simulink model "Milestone_2_Hardware"  (R2021a)
settings: Solver=FixedStepDiscrete  StartTime=0.0  StopTime=10  FixedStep=0.01  RelTol=1e-3  EnableMultiTasking=on
values from neighbouring files (symbols this model uses):
  ticksPerRot =     [robotParameters.m]
  wheelR =     [robotParameters.m]
undefined symbols (not defined in the file or in its folder): InputPWM, WheelSpeed
libraries: arduinolib x10, spsEdgeDetectorLib x2, pid_lib x2, mobileRoboticsTrainingLib x1
settings Model: SILPILModeSetting=veronly  ExtModeTrigDuration=2  Creator=Boitumelo  LastModifiedBy=brennannaidoo
settings OptimizationCC: EnhancedBackFolding=on  PassReuseOutputArgsAs=Individual arguments  ZeroExternalMemoryAtStartup=off  ZeroInternalMemoryAtStartup=off  MaxStackSize=64  OptimizeBlockOrder=speed  DifferentSizesBufferReuse=on  OptimizationCustomize=off  EfficientTunableParamExpr=on
settings DebuggingCC: ParameterTunabilityLossMsg=error
settings HardwareCC: ProdBitPerInt=16  ProdBitPerPointer=16  ProdBitPerSizeT=16  ProdBitPerPtrDiffT=16  ProdLargestAtomicFloat=None  ProdWordSize=8  ProdHWDeviceType=Atmel->AVR  UseEmbeddedCoderFeatures=off  UseSimulinkCoderFeatures=off
settings SFSimCC: MATLABDynamicMemAlloc=off
settings RTWCC: SystemTargetFile=ert.tlc  HardwareBoard=Arduino Uno  TemplateMakefile=ert_default_tmf  Toolchain=Arduino AVR  BuildConfiguration=Faster Runs
settings CodeAppCC: ForceParamTrailComments=on  IgnoreCustomStorageClasses=off  OperatorAnnotations=on  SimulinkDataObjDesc=on  SFDataObjDesc=on  InsertBlockDesc=on
settings ERTTargetCC: SupportContinuousTime=on  SupportNonInlinedSFcns=on  SupportVariableSizeSignals=on  ExtModeStaticAllocSize=250

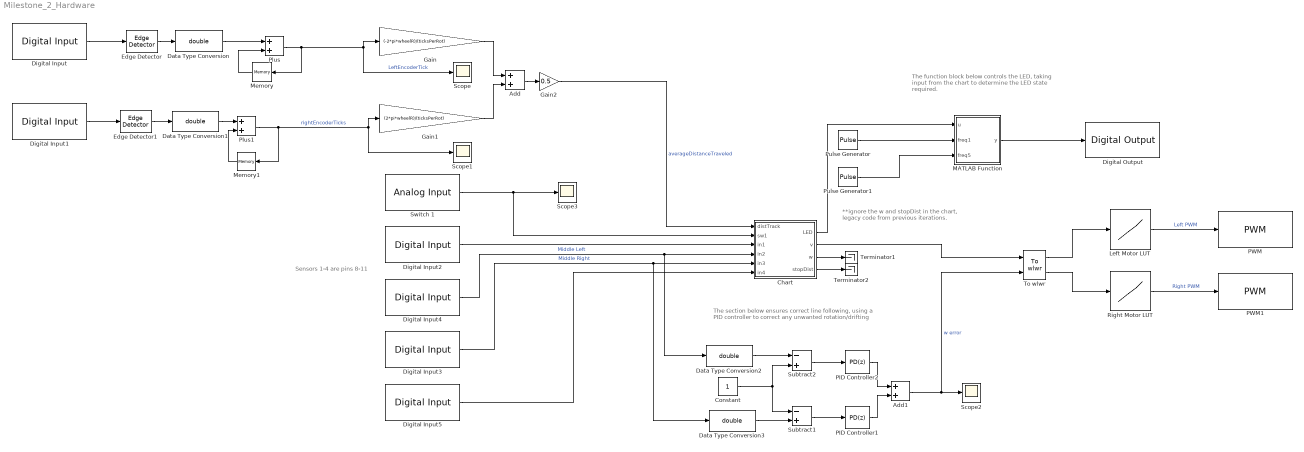
== system Milestone_2_Hardware ==
  note: Sensors 1-4 are pins 8-11
  note: **ignore the w and stopDist in the chart, legacy code from previous iterations.
  note: The section below ensures correct line following, using a PID controller to correct any unwanted rotation/drifting
  note: The function block below controls the LED, taking input from the chart to determine the LED state required.
  Add : Sum
  Add1 : Sum
  Chart : Stateflow chart  TreatAsAtomicUnit=on
      settings: PortSchema="{\"entries\":[{\"content\":{\"sides\":[{\"content\":{\"connectorIds\":[\"In1\",\"In2\",\"In3\",\"In4\",\"In5\",\"In6\"]},\"type\":\"ConnectorPlacement.EquallySpacedRectSide\",\"uuid\":\"78c7eb26-8bbd-447d-a092-1af712c17389\"},{\"content\":{\"connectorIds\":[\"Out1\",\"Out3\",\"Out4\",\"Out2\"],\"side\":\"RIGHT\"},\"type\":\"ConnectorPlacement.EquallySpacedRectSide\",\"uuid\":\"da6b3332-17f7-4001-b928-64a5d6ce29c5\"},{\"content\":{\"connectorIds\":[],\"side\":\"TOP\"},\"type\":\"ConnectorPlacement.EquallySpacedRectSide\",\"uuid\":\"abb817b7-61f9-479c-a331-9ffc37da7474\"},{\"content\":{\"connectorIds\":[],\"side\":\"BOTTOM\"},\"type\":\"ConnectorPlacement.EquallySpacedRectSide\",\"uuid\":\"3a592b8d-4d7e-4d46-b4df-a225774e50cb\"}]},\"type\":\"ConnectorPlacement.EquallySpacedConnector\",\"uuid\":\"ef174e7d-a0f4-4cd7-8d3f-242f6d04d2d1\"}],\"packageUris\":[\"http://schema.mathworks.com/mf0/Connector/R2020b\"],\"version\":\"1.0\"}"
  Constant : Constant
  Data Type Conversion{,1..3} (4 alike) : DataTypeConversion  OutDataTypeStr=double
  Digital Input : arduinolib/Digital Input  pinNumber=2  mode=Default  Direction=input  SampleTime=0.01  blockPlatform=arduino
  Digital Input1 : arduinolib/Digital Input  pinNumber=3  mode=Default  Direction=input  SampleTime=0.01  blockPlatform=arduino
  Digital Input2 : arduinolib/Digital Input  pinNumber=8  mode=Default  Direction=input  SampleTime=0.01  blockPlatform=arduino
  Digital Input3 : arduinolib/Digital Input  pinNumber=10  mode=Default  Direction=input  SampleTime=0.01  blockPlatform=arduino
  Digital Input4 : arduinolib/Digital Input  pinNumber=9  mode=Default  Direction=input  SampleTime=0.01  blockPlatform=arduino
  Digital Input5 : arduinolib/Digital Input  pinNumber=11  mode=Default  Direction=input  SampleTime=0.01  blockPlatform=arduino
  Digital Output : arduinolib/Digital Output  pinNumber=13  Direction=output  blockPlatform=arduino
  Edge Detector : spsEdgeDetectorLib/Edge Detector  model=Either  ic=0  Ts=0
      settings: SourceProductBaseCode=PS
  Edge Detector1 : spsEdgeDetectorLib/Edge Detector  model=Either  ic=0  Ts=0
      settings: SourceProductBaseCode=PS
  Gain : Gain  Gain=(-2*pi*wheelR)/(ticksPerRot)
  Gain1 : Gain  Gain=(2*pi*wheelR)/(ticksPerRot)
  Gain2 : Gain  Gain=0.5
  Left Motor LUT : Lookup_n-D  NumberOfTableDimensions=1  BreakpointsForDimension1=WheelSpeed  Table=InputPWM  InterpMethod=Nearest  ExtrapMethod=Clip  InternalRulePriority=Speed  RndMeth=Simplest  InputSameDT=on
  MATLAB Function : MATLAB Function  TreatAsAtomicUnit=on
  Memory : Memory
  Memory1 : Memory
  PID Controller1 : pid_lib/PID Controller  Controller=PD  Form=Parallel  TimeDomain=Discrete-time  UseExternalTs=off  SampleTime=-1  IntegratorMethod=Forward Euler  FilterMethod=Forward Euler  ControllerParametersSource=internal  P=1  I=1  D=1e-5  UseFilter=on  N=100  TunerSelectOption=Transfer Function Based (PID Tuner App)  InitialConditionSource=internal  InitialConditionForIntegrator=0  InitialConditionForFilter=0  DifferentiatorICPrevScaledInput=0  ExternalReset=none  TrackingMode=off  Kt=1  LimitOutput=off  SatLimitsSource=internal  UpperSaturationLimit=inf  LowerSaturationLimit=-inf  LinearizeAsGain=on  AntiWindupMode=none  Kb=1  POutMin=[]  POutMax=[]  IOutMin=[]  IOutMax=[]  DOutMin=[]  DOutMax=[]  NOutMin=[]  NOutMax=[]  SumOutMin=[]  SumOutMax=[]  SaturationOutMin=[]  SaturationOutMax=[]  PParamMin=[]  PParamMax=[]  IParamMin=[]  IParamMax=[]  DParamMin=[]  DParamMax=[]  NParamMin=[]  NParamMax=[]  KbParamMin=[]  KbParamMax=[]  KtParamMin=[]  KtParamMax=[]  KbOutMin=[]  KbOutMax=[]  KtOutMin=[]  KtOutMax=[]  IntegratorOutMin=[]  IntegratorOutMax=[]  FilterOutMin=[]  FilterOutMax=[]  SumI1OutMin=[]  SumI1OutMax=[]  SumI2OutMin=[]  SumI2OutMax=[]  SumI3OutMin=[]  SumI3OutMax=[]  SumI4OutMin=[]  SumI4OutMax=[]  SumDOutMin=[]  SumDOutMax=[]  DifferentiatorOutMin=[]  DifferentiatorOutMax=[]  FilterDiffOutCoefMin=[]  FilterDiffOutCoefMax=[]  ReciprocalOutMin=[]  ReciprocalOutMax=[]  SumDenOutMin=[]  SumDenOutMax=[]  SumNumOutMin=[]  SumNumOutMax=[]  DivideOutMin=[]  DivideOutMax=[]  UdiffTsProdOutMin=[]  UdiffTsProdOutMax=[]  NTsProdOutMin=[]  NTsProdOutMax=[]  UintegralTsProdOutMin=[]  UintegralTsProdOutMax=[]  UngainTsProdOutMin=[]  UngainTsProdOutMax=[]  IntegratorContinuousStateAttributes=''  IntegratorStateMustResolveToSignalObject=off  IntegratorRTWStateStorageClass=Auto  FilterContinuousStateAttributes=''  FilterStateMustResolveToSignalObject=off  FilterRTWStateStorageClass=Auto  ParallelPVariant=InternalParameters  IdealPVariant=Disabled  IVariant=Disabled  DVariant=InternalParameters  IntegratorVariant=Disabled  SatVariant=Disabled  AWVariant=Disabled  PCopyVariant=Disabled  TRVariant=Disabled  FdbkBlocksVariant=Forward  IdealPFdbkVariant=Disabled  SatFdbkVariant=Disabled  DerivativeFilterVariant=ForwardEulerFilter  NVariant=InternalParameters  NCopyVariant=Disabled  FilterICVariant=InternalICsFilter  IntegratorICVariant=Disabled  ExternalResetVariant=Disabled  TRSumVariant=Passthrough  SumFdbkVariant=Disabled  SumVariant=Sum_PD  TsampFilterVariant=InternalTs  TsampNgainVariant=Passthrough  TsampIntegralVariant=Disabled_SignalSpec  ExternalSaturationOutDataTypeStr=Inherit: Same as second input  InitialConditionSetting=Output
  PID Controller2 : pid_lib/PID Controller  Controller=PD  Form=Parallel  TimeDomain=Discrete-time  UseExternalTs=off  SampleTime=-1  IntegratorMethod=Forward Euler  FilterMethod=Forward Euler  ControllerParametersSource=internal  P=1  I=1  D=1e-5  UseFilter=on  N=100  TunerSelectOption=Transfer Function Based (PID Tuner App)  InitialConditionSource=internal  InitialConditionForIntegrator=0  InitialConditionForFilter=0  DifferentiatorICPrevScaledInput=0  ExternalReset=none  TrackingMode=off  Kt=1  LimitOutput=off  SatLimitsSource=internal  UpperSaturationLimit=inf  LowerSaturationLimit=-inf  LinearizeAsGain=on  AntiWindupMode=none  Kb=1  POutMin=[]  POutMax=[]  IOutMin=[]  IOutMax=[]  DOutMin=[]  DOutMax=[]  NOutMin=[]  NOutMax=[]  SumOutMin=[]  SumOutMax=[]  SaturationOutMin=[]  SaturationOutMax=[]  PParamMin=[]  PParamMax=[]  IParamMin=[]  IParamMax=[]  DParamMin=[]  DParamMax=[]  NParamMin=[]  NParamMax=[]  KbParamMin=[]  KbParamMax=[]  KtParamMin=[]  KtParamMax=[]  KbOutMin=[]  KbOutMax=[]  KtOutMin=[]  KtOutMax=[]  IntegratorOutMin=[]  IntegratorOutMax=[]  FilterOutMin=[]  FilterOutMax=[]  SumI1OutMin=[]  SumI1OutMax=[]  SumI2OutMin=[]  SumI2OutMax=[]  SumI3OutMin=[]  SumI3OutMax=[]  SumI4OutMin=[]  SumI4OutMax=[]  SumDOutMin=[]  SumDOutMax=[]  DifferentiatorOutMin=[]  DifferentiatorOutMax=[]  FilterDiffOutCoefMin=[]  FilterDiffOutCoefMax=[]  ReciprocalOutMin=[]  ReciprocalOutMax=[]  SumDenOutMin=[]  SumDenOutMax=[]  SumNumOutMin=[]  SumNumOutMax=[]  DivideOutMin=[]  DivideOutMax=[]  UdiffTsProdOutMin=[]  UdiffTsProdOutMax=[]  NTsProdOutMin=[]  NTsProdOutMax=[]  UintegralTsProdOutMin=[]  UintegralTsProdOutMax=[]  UngainTsProdOutMin=[]  UngainTsProdOutMax=[]  IntegratorContinuousStateAttributes=''  IntegratorStateMustResolveToSignalObject=off  IntegratorRTWStateStorageClass=Auto  FilterContinuousStateAttributes=''  FilterStateMustResolveToSignalObject=off  FilterRTWStateStorageClass=Auto  ParallelPVariant=InternalParameters  IdealPVariant=Disabled  IVariant=Disabled  DVariant=InternalParameters  IntegratorVariant=Disabled  SatVariant=Disabled  AWVariant=Disabled  PCopyVariant=Disabled  TRVariant=Disabled  FdbkBlocksVariant=Forward  IdealPFdbkVariant=Disabled  SatFdbkVariant=Disabled  DerivativeFilterVariant=ForwardEulerFilter  NVariant=InternalParameters  NCopyVariant=Disabled  FilterICVariant=InternalICsFilter  IntegratorICVariant=Disabled  ExternalResetVariant=Disabled  TRSumVariant=Passthrough  SumFdbkVariant=Disabled  SumVariant=Sum_PD  TsampFilterVariant=InternalTs  TsampNgainVariant=Passthrough  TsampIntegralVariant=Disabled_SignalSpec  ExternalSaturationOutDataTypeStr=Inherit: Same as second input  InitialConditionSetting=Output
  PWM : arduinolib/PWM  pinNumber=5  frequencyType=Default  desiredFrequency=490.2  achievableFrequency=490.2
  PWM1 : arduinolib/PWM  pinNumber=6  frequencyType=Default  desiredFrequency=490.2  achievableFrequency=490.2
  Plus : Sum
  Plus1 : Sum
  Pulse Generator : DiscretePulseGenerator  PulseType=Time based  PulseWidth=50
  Pulse Generator1 : DiscretePulseGenerator  PulseType=Time based  Period=0.4  PulseWidth=50
  Right Motor LUT : Lookup_n-D  NumberOfTableDimensions=1  BreakpointsForDimension1=WheelSpeed  Table=InputPWM  InterpMethod=Nearest  ExtrapMethod=Clip  InternalRulePriority=Speed  RndMeth=Simplest  InputSameDT=on
  Scope{,1..3} (4 alike) : Scope
  Subtract1 : Sum  Inputs=-+
  Subtract2 : Sum  Inputs=-+
  Switch 1 : arduinolib/Analog Input  pinNumber=0  ReadResultsOnly=off  ConversionTriggerSource=Software  ExternalTriggerType=uint32( 0 )  OutputDataType=uint16  EnableConversionCompleteNotify=off  EnableOuputStatus=off  SampleTime=0.01  blockPlatform=arduino
  Terminator1 : Terminator
  Terminator2 : Terminator
  To wlwr : mobileRoboticsTrainingLib/To wlwr  axleLength=0.1  wheelR=0.05
  wires:
  Right Motor LUT/1 -> PWM1/1  "Right PWM"
  Left Motor LUT/1 -> PWM/1  "Left PWM"
  To wlwr/1 -> Left Motor LUT/1
  To wlwr/2 -> Right Motor LUT/1
  Add/1 -> Gain2/1
  Gain/1 -> Add/1
  Gain1/1 -> Add/2
  Gain2/1 -> Chart/1(distTrack)  "averageDistanceTraveled"
  Edge Detector1/1 -> Data Type Conversion1/1
  Digital Input1/1 -> Edge Detector1/1
  Plus1/1 -> Memory1/1, Scope1/1, Gain1/1  "rightEncoderTicks"
  Memory1/1 -> Plus1/2
  Data Type Conversion1/1 -> Plus1/1
  Data Type Conversion/1 -> Plus/1
  Edge Detector/1 -> Data Type Conversion/1
  Plus/1 -> Memory/1, Scope/1, Gain/1  "LeftEncoderTick"
  Digital Input/1 -> Edge Detector/1
  Memory/1 -> Plus/2
  Digital Input2/1 -> Chart/3(in1)
  Digital Input4/1 -> Data Type Conversion2/1, Chart/4(in2)  "Middle Left"
  Digital Input3/1 -> Chart/5(in3), Data Type Conversion3/1  "Middle Right"
  Digital Input5/1 -> Chart/6(in4)
  Chart/4(w) -> Terminator1/1
  Chart/3(v) -> To wlwr/1
  Subtract1/1 -> PID Controller1/1
  Add1/1 -> To wlwr/2, Scope2/1  "w error"
  Data Type Conversion2/1 -> Subtract2/1
  Data Type Conversion3/1 -> Subtract1/2
  Switch 1/1 -> Chart/2(sw1), Scope3/1
  Subtract2/1 -> PID Controller2/1
  Constant/1 -> Subtract2/2, Subtract1/1
  PID Controller1/1 -> Add1/2
  PID Controller2/1 -> Add1/1
  Chart/1(LED) -> MATLAB Function/1(u)
  Pulse Generator/1 -> MATLAB Function/2(freq1)
  Pulse Generator1/1 -> MATLAB Function/3(freq5)
  MATLAB Function/1(y) -> Digital Output/1
  Chart/2(stopDist) -> Terminator2/1

== matlab function Milestone_2_Hardware/MATLAB Function ==
  data: u input; y output; freq1 input; freq5 input
function y = fcn(u,freq1, freq5)
    if u==0
        y=0;
    elseif u==1
        y=freq1;
    elseif u==5
        y=freq5;
    else 
        y=1;
    end

== stateflow chart Milestone_2_Hardware/Chart ==
  state DeadEnd
    entry:
    v=0;
    w=0;
    LED=10
  state CrossRoads
    entry:
    v=0;
    w=0
    LED=10;
  state Junction1_0000_
    entry:
    v=0.1;
    w=0;
    stopDist=0.065
    LED=5
    startDist = distTrack
  note: distTrack ensures the sensors pass the junction before taking the final reading. This is necessary to prevent incorrect junction detection.
  state Initial
    entry:
    v=0;
    w=0;
    stopDist=0
    LED=0
  state MoveForward
    v=0.1;
    w=0;
    stopDist=2
    LED=1
  state TJunc
    entry:
    v=0;
    w=0;
    LED = 10
  state StartDetect
    entry:
    stopDist=0
  state Junction2_1000_
    entry:
    v=0.1;
    w=0;
    stopDist=0.018
    LED=5
    startDist = distTrack
  state RightTurn
    entry:
    v=0;
    w=0;
    LED=10
  state RightTJunc
    entry:
    v=0;
    w=0;
    LED=10
  state Junction3_0001_
    entry:
    v=0.1;
    w=0;
    stopDist=0.018
    LED=5
    startDist = distTrack
  state LeftTurn
    entry:
    v=0;
    w=0;
    LED=10
  state LeftTJunc
    entry:
    v=0;
    w=0;
    LED=10
  state DeadEnd1
    entry:
    v=0;
    w=0;
    LED=10
  Junction1_0000_ -> DeadEnd [order 1] : [distTrack >= (startDist + 0.050) & in1==0 & in2==0 & in3==0 & in4==0 ]
  Junction1_0000_ -> CrossRoads [order 2] : [distTrack >= (startDist + 0.050) & in1==1 & in2==0 & in3==0 & in4==1 ]
  MoveForward -> Junction1_0000_ [order 1] : [in1==0 & in2==0 & in3==0 & in4==0 ]
  (default) -> Initial
  Junction1_0000_ -> TJunc [order 3] : [distTrack >= (startDist + 0.050) & in1==1 & in2==1 & in3==1 & in4==1 ]
  StartDetect -> MoveForward : [in2==0 & in3==0]
  Initial -> StartDetect : [sw1==0]
  MoveForward -> Junction2_1000_ [order 2] : [in1==1 & in2==0 & in3==0 & in4==0]
  MoveForward -> DeadEnd1 [order 4] : [in1==1 & in2==1 & in3==1 & in4==1]
  MoveForward -> Junction3_0001_ [order 3] : [in1==0 & in2==0 & in3==0 & in4==1]
  Junction2_1000_ -> RightTurn [order 1] : [distTrack >= (startDist + 0.050) & in1==1 & in2==1 & in3==1 & in4==1 ]
  Junction2_1000_ -> RightTJunc [order 2] : [distTrack >= (startDist + 0.050) & in1==1 & in2==0 & in3==0 & in4==1 ]
  Junction3_0001_ -> LeftTurn [order 1] : [distTrack >= (startDist + 0.050) & in1==in2==in3==in4==1]
  Junction3_0001_ -> LeftTJunc [order 2] : [distTrack >= (startDist + 0.050) & in1==1 & in2==0 & in3==0 & in4==1 ]
  data: LED output; distTrack input; sw1 input; stopDist output; in1 input; in2 input; in3 input; in4 input; v output; w output; startDist local
